simulink model "Project3Week1_notireslip"  (R2024b)
settings: Solver=VariableStepAuto  StartTime=0.0  StopTime=765  RelTol=1e-3
values from neighbouring files (symbols this model uses):
  ad = 2.25    [Project3Week1.m]
  b_capacity = 50    [Project3Week1.m]
  cd = 0.34    [Project3Week1.m]
  eta_motor = 0.9    [Project3Week1.m]
  gratio = 2    [Project3Week1.m]
  i_gear_i = 0.5    [Project3Week1.m]
  ipt = 10    [Project3Week1.m]
  iw = 9    [Project3Week1.m]
  kd = .005    (= 0.005)    [Project3Week1.m]
  ki = .02    (= 0.02)    [Project3Week1.m]
  kp = 0.0075    [Project3Week1.m]
  l_time = l_time(2:end)    [Project3Week1.m]
  l_vel = l_vel(2:end) * 0.44704    [Project3Week1.m]
  motor_torque_curve = [motor_rpm', motor_torque']    [Project3Week1.m]
  o_gear_i = 0.7    [Project3Week1.m]
  r_internal = 0.05    [Project3Week1.m]
  rho = 1.293    [Project3Week1.m]
  rw = 0.48/2    (= 0.24)    [Project3Week1.m]
  soc_min = 0.1    [Project3Week1.m]
  tau_brakes = 1500    [Project3Week1.m]
  v_batt = 350    [Project3Week1.m]
  vm = 1600    [Project3Week1.m]
settings Model: Creator=btagl  LastModifiedBy=btagl

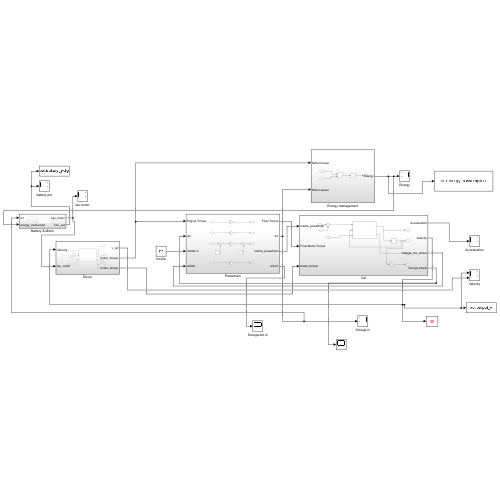
[thumbnail: Simulink's stored preview of the top-level diagram]
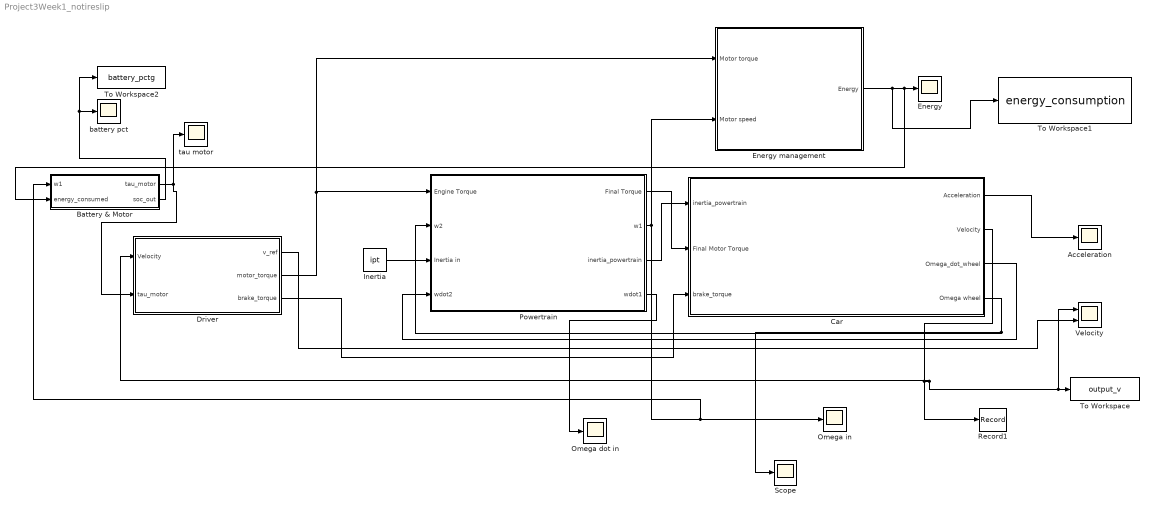
== system Project3Week1_notireslip ==
  Acceleration : Scope
  Battery & Motor : Subsystem
  Car : Subsystem
  Driver : Subsystem
  Energy : Scope
  Energy management : Subsystem
  Inertia : Constant  Value=ipt
  Omega dot in : Scope
  Omega in : Scope
  Powertrain : Subsystem
  Record1 : Record  VariableName=actual_v  RecordToWorkspace=on  FileSettingsInternal="{\"entries\":[{\"content\":{\"excelSettings\":{\"content\":{},\"type\":\"Streamout.ExcelSettings\"}},\"type\":\"Streamout.FileSettingStorage\",\"uuid\":\"\"}],\"packageUris\":[\"http:\\/\\/schema.mathworks.com\\/mf0\\/streamout_blocks\\/R2020a\"],\"version\":\"1.0\"}"  SignalsInternal="{\"entries\":[{\"content\":{\"signals\":[{\"content\":{\"blockPath\":[],\"dimensions\":[1],\"domain\":\"\",\"lineColor\":\"#4dbeee\",\"lineWidth\":2,\"plots\":[ 1 ],\"port\":1,\"sid\":[\"\"],\"signalID\":1,\"signalName\":\"Car:2\"},\"type\":\"RecordBlkView.Signal\",\"uuid\":\"\"}]},\"type\":\"RecordBlkView.InputSignals\",\"uuid\":\"\"}],\"packageUris\":[\"http:\\/\\/schema.mathworks.com\\/mf0\\/streamout_blocks\\/R2020a\"],\"version\":\"1.0\"}"  VisualizationBindings="{\"sparklinesplugin\":{\"info\":[{\"bindingParametersList\":[],\"subplotID\":1}]}}"
  Scope : Scope
  To Workspace : ToWorkspace  VariableName=output_v  SampleTime=-1
  To Workspace1 : ToWorkspace  VariableName=energy_consumption  SaveFormat=Timeseries  SampleTime=-1
  To Workspace2 : ToWorkspace  VariableName=battery_pctg  SaveFormat=Timeseries  SampleTime=-1
  Velocity : Scope  NumInputPorts=2
  battery pct : Scope
  tau motor : Scope
  wires:
  Car/2(Velocity) -> Velocity/1, To Workspace/1, Driver/1(Velocity), Record1/1
  Car/1(Acceleration) -> Acceleration/1
  Driver/1(v_ref) -> Velocity/2
  Powertrain/3(inertia_powertrain) -> Car/1(inertia_powertrain)
  Inertia/1 -> Powertrain/3(Inertia in)
  Car/4(Omega wheel) -> Scope/1, Powertrain/2(w2)
  Powertrain/4(wdot1) -> Omega dot in/1
  Car/3(Omega_dot_wheel) -> Powertrain/4(wdot2)
  Energy management/1(Energy) -> To Workspace1/1, Battery & Motor/2(energy_consumed), Energy/1
  Driver/2(motor_torque) -> Energy management/1(Motor torque), Powertrain/1(Engine Torque)
  Powertrain/1(Final Torque) -> Car/2(Final Motor Torque)
  Driver/3(brake_torque) -> Car/3(brake_torque)
  Powertrain/2(w1) -> Battery & Motor/1(w1), Omega in/1, Energy management/2(Motor speed)
  Battery & Motor/1(tau_motor) -> Driver/2(tau_motor), tau motor/1
  Battery & Motor/2(soc_out) -> To Workspace2/1, battery pct/1

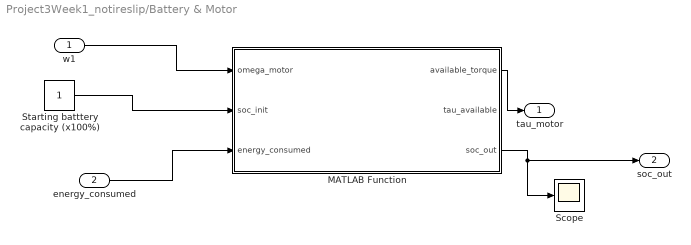
== system Project3Week1_notireslip/Battery & Motor ==
  w1 : Inport
  energy_consumed : Inport  Port=2
  MATLAB Function : MATLAB Function  TreatAsAtomicUnit=on
  Scope : Scope
  Starting batttery capacity (x100%) : Constant
  tau_motor : Outport
  soc_out : Outport  Port=2
  wires:
  MATLAB Function/1(available_torque) -> tau_motor/1
  w1/1 -> MATLAB Function/1(omega_motor)
  Starting batttery capacity (x100%)/1 -> MATLAB Function/2(soc_init)
  energy_consumed/1 -> MATLAB Function/3(energy_consumed)
  MATLAB Function/3(soc_out) -> soc_out/1, Scope/1

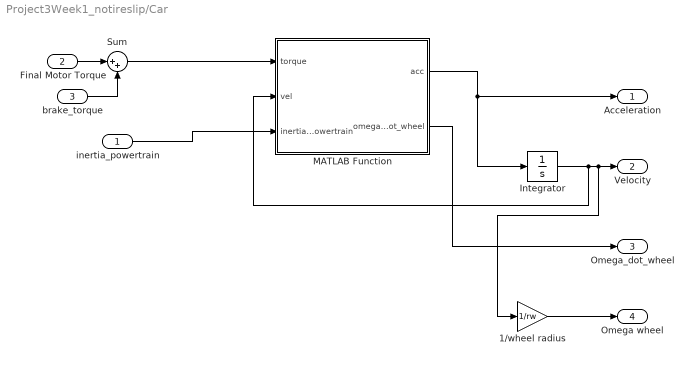
== system Project3Week1_notireslip/Car ==
  inertia_powertrain : Inport
  Final Motor Torque : Inport  Port=2
  brake_torque : Inport  Port=3
  1/wheel radius : Gain  Gain=1/rw
  Integrator : Integrator
  MATLAB Function : MATLAB Function  TreatAsAtomicUnit=on
  Sum : Sum  Inputs=|++
  Acceleration : Outport
  Velocity : Outport  Port=2
  Omega_dot_wheel : Outport  Port=3
  Omega wheel : Outport  Port=4
  wires:
  Sum/1 -> MATLAB Function/1(torque)
  MATLAB Function/1(acc) -> Integrator/1, Acceleration/1
  Integrator/1 -> MATLAB Function/2(vel), 1/wheel radius/1, Velocity/1
  inertia_powertrain/1 -> MATLAB Function/3(inertia_powertrain)
  MATLAB Function/2(omega_dot_wheel) -> Omega_dot_wheel/1
  1/wheel radius/1 -> Omega wheel/1
  Final Motor Torque/1 -> Sum/1
  brake_torque/1 -> Sum/2

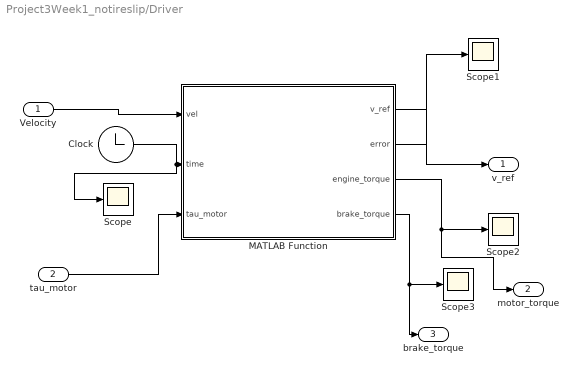
== system Project3Week1_notireslip/Driver ==
  Velocity : Inport
  tau_motor : Inport  Port=2
  Clock : Clock
  MATLAB Function : MATLAB Function  TreatAsAtomicUnit=on
  Scope{,1..3} (4 alike) : Scope
  v_ref : Outport
  motor_torque : Outport  Port=2
  brake_torque : Outport  Port=3
  wires:
  Velocity/1 -> MATLAB Function/1(vel)
  Clock/1 -> Scope/1, MATLAB Function/2(time)
  MATLAB Function/1(v_ref) -> v_ref/1
  MATLAB Function/2(error) -> Scope1/1
  MATLAB Function/3(engine_torque) -> motor_torque/1, Scope2/1
  MATLAB Function/4(brake_torque) -> brake_torque/1, Scope3/1
  tau_motor/1 -> MATLAB Function/3(tau_motor)

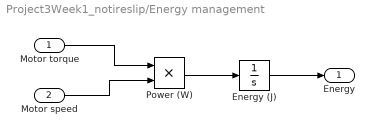
== system Project3Week1_notireslip/Energy management ==
  Motor torque : Inport
  Motor speed : Inport  Port=2
  Energy (J) : Integrator
  Power (W) : Product
  Energy : Outport
  wires:
  Motor torque/1 -> Power (W)/1
  Motor speed/1 -> Power (W)/2
  Power (W)/1 -> Energy (J)/1
  Energy (J)/1 -> Energy/1

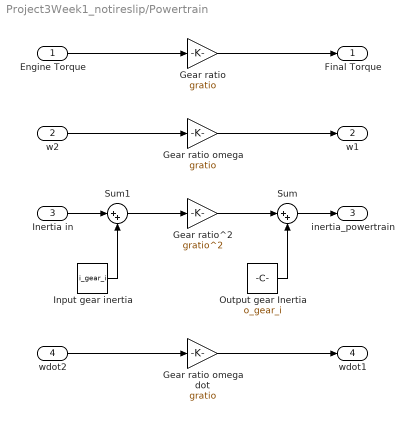
== system Project3Week1_notireslip/Powertrain ==
  Engine Torque : Inport
  w2 : Inport  Port=2
  Inertia in : Inport  Port=3
  wdot2 : Inport  Port=4
  Gear ratio : Gain  Gain=gratio
  Gear ratio omega : Gain  Gain=gratio
  Gear ratio omega dot : Gain  Gain=gratio
  Gear ratio^2 : Gain  Gain=gratio^2
  Input gear inertia : Constant  Value=i_gear_i
  Output gear Inertia : Constant  Value=o_gear_i
  Sum : Sum  Inputs=|++
  Sum1 : Sum  Inputs=|++
  Final Torque : Outport
  w1 : Outport  Port=2
  inertia_powertrain : Outport  Port=3
  wdot1 : Outport  Port=4
  wires:
  Engine Torque/1 -> Gear ratio/1
  Gear ratio/1 -> Final Torque/1
  Gear ratio omega/1 -> w1/1
  w2/1 -> Gear ratio omega/1
  Input gear inertia/1 -> Sum1/2
  Inertia in/1 -> Sum1/1
  Sum1/1 -> Gear ratio^2/1
  Output gear Inertia/1 -> Sum/2
  Gear ratio^2/1 -> Sum/1
  Sum/1 -> inertia_powertrain/1
  Gear ratio omega dot/1 -> wdot1/1
  wdot2/1 -> Gear ratio omega dot/1

== matlab function Project3Week1_notireslip/Driver/MATLAB Function ==
  settings: updateMethod=DISCRETE  sampleTime=0.001
  data: vel input; time input; l_time parameter; l_vel parameter; kp parameter; ki parameter; kd parameter; v_ref output; error output; tau_brakes parameter; engine_torque output; brake_torque output; tau_motor input
function [v_ref, error, engine_torque, brake_torque] = driver_model(...
    vel, time, l_time, l_vel, kp, ki, kd, tau_brakes, tau_motor)
    tau_regen_max=tau_motor*0.6;
    % Persistent variables for integral and previous error
    persistent integral_error prev_error;
    if isempty(integral_error)
        integral_error = 0;
        prev_error = 0;
    end

    % Reference velocity
    v_ref = interp1(l_time, l_vel, time, 'linear', 'extrap');
    error = v_ref - vel;

    % PID Control
    integral_error = integral_error + error;
    derivative_error = error - prev_error;
    prev_error = error;

    % Control signal (alpha)
    alpha_driver = kp * error + ki * integral_error + kd * derivative_error;
    alpha_driver = max(-1, min(1, alpha_driver));

    % Torque calculation
    if alpha_driver >= 0
        % Acceleration phase
        engine_torque = alpha_driver * tau_motor;
        brake_torque = 0;
    else
        % Deceleration phase: regen + friction
        brake_torque_total = -alpha_driver * tau_brakes;

        % Limit regen to tau_regen_max
        regen_torque = min(brake_torque_total, tau_regen_max);

        % Apply regen as negative motor torque
        engine_torque = -regen_torque;

        % Remaining torque goes to brakes
        brake_torque = -(brake_torque_total - regen_torque);
    end
end

== matlab function Project3Week1_notireslip/Car/MATLAB Function ==
  data: acc output; torque input; iw parameter; rw parameter; vm parameter; cd parameter; vel input; ad parameter; rho parameter; inertia_powertrain input; omega_dot_wheel output
function [acc, omega_dot_wheel] = fcn(torque, iw, rw, vm, cd,vel,ad,rho, inertia_powertrain)

fdrag=0.5*(rho*ad*cd*vel^2);
meq=((inertia_powertrain+iw)/rw^2)+vm;
fx=(torque/rw)-fdrag;
acc=(fx/meq);
omega_dot_wheel=acc/rw; %rad/s^2 angular acceleration

== matlab function Project3Week1_notireslip/Battery & Motor/MATLAB Function ==
  data: omega_motor input; v_batt parameter; r_internal parameter; eta_motor parameter; soc_min parameter; soc_init input; motor_torque_curve parameter; available_torque output; tau_available output; energy_consumed input; soc_out output; b_capacity parameter
function [available_torque, tau_available, soc_out] = compute_available_torque(...
    omega_motor, v_batt, r_internal, eta_motor, soc_min, soc_init, ...
    motor_torque_curve, energy_consumed, b_capacity)

    % Convert omega (rad/s) to RPM
    rpm_motor = omega_motor * 60 / (2 * pi);

    % Lookup motor torque limit at current RPM
    tau_motor_limit = interp1(motor_torque_curve(:,1), motor_torque_curve(:,2), ...
                              rpm_motor, 'linear', 'extrap');

    % Compute SOC based on energy used so far
    soc_out = soc_init - (energy_consumed / (3600 * v_batt * b_capacity));
    soc_out = max(soc_min, soc_out);  % prevent dropping below min

    % Default torque values
    available_torque = 0;
    tau_available = 0;

    % Case 1: SOC too low
    if soc_out <= soc_min
        return;

    % Case 2: Motor is stalled
    elseif omega_motor < 1e-3
        available_torque = tau_motor_limit;
        tau_available = available_torque;

    % Case 3: Power-limited torque
    else
        p_max_batt = (v_batt^2) / (4 * r_internal);
        p_mech_available = p_max_batt * eta_motor;
        tau_available_batt = p_mech_available / omega_motor;

        % Final torque = limited by both motor and battery
        available_torque = min(tau_available_batt, tau_motor_limit);
        tau_available = tau_available_batt;
    end
end
